simulink model "Serial_Com_Ex"  (R2022b)
settings: Solver=VariableStepAuto  StartTime=0.0  StopTime=10.0  RelTol=1e-3
libraries: etargetslib x4, frdmk64flib x2
settings Model: Creator=samcr  LastModifiedBy=samcr

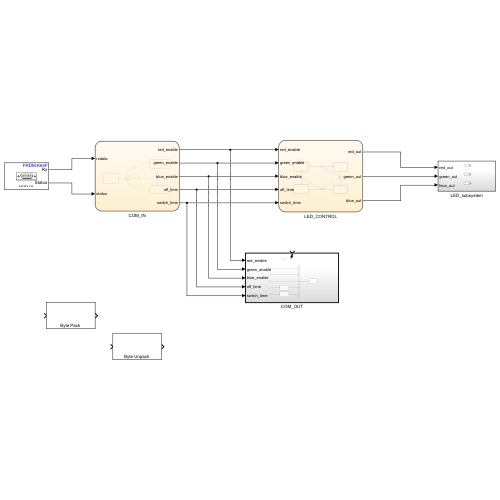
[thumbnail: Simulink's stored preview of the top-level diagram]
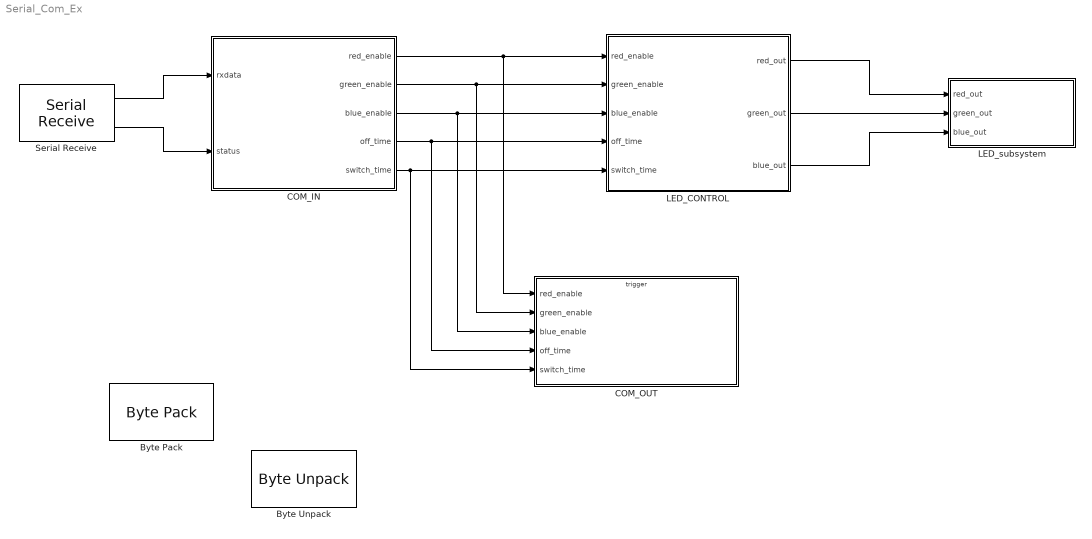
== system Serial_Com_Ex ==
  Byte Pack : etargetslib/Byte Pack  datatypes={'double'}  byteAlign=1
  Byte Unpack : etargetslib/Byte Unpack  dimensions={[1]}  datatypes={'double'}  byteAlign=1
      settings: LibrarySourceBlock=embeddedtargetslib/Host Communication/Byte Unpack
  COM_IN : Stateflow chart  TreatAsAtomicUnit=on
  COM_OUT : Subsystem
  LED_CONTROL : Stateflow chart  TreatAsAtomicUnit=on
  LED_subsystem : Subsystem
  Serial Receive : frdmk64flib/Serial Receive  SCIModule=0  Baudrate=uint32(9600)  Parity=None  StopBits=1  HardwareFlowControl=None  ByteOrder=LittleEndian  DataType=uint8  DataLength=10  BlockingMode=off  OutputStatus=on  SampleTime=-1
  wires:
  Serial Receive/1 -> COM_IN/1(rxdata)
  Serial Receive/2 -> COM_IN/2(status)
  COM_IN/1(red_enable) -> COM_OUT/1(red_enable), LED_CONTROL/1(red_enable)
  COM_IN/2(green_enable) -> COM_OUT/2(green_enable), LED_CONTROL/2(green_enable)
  COM_IN/3(blue_enable) -> COM_OUT/3(blue_enable), LED_CONTROL/3(blue_enable)
  COM_IN/4(off_time) -> COM_OUT/4(off_time), LED_CONTROL/4(off_time)
  COM_IN/5(switch_time) -> LED_CONTROL/5(switch_time), COM_OUT/5(switch_time)
  LED_CONTROL/2(green_out) -> LED_subsystem/2(green_out)
  LED_CONTROL/3(blue_out) -> LED_subsystem/3(blue_out)
  LED_CONTROL/1(red_out) -> LED_subsystem/1(red_out)

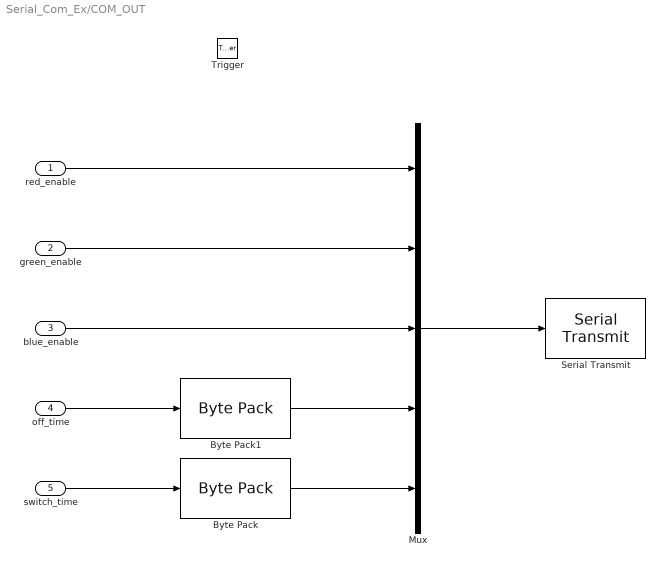
== system Serial_Com_Ex/COM_OUT ==
  red_enable : Inport
  green_enable : Inport  Port=2
  blue_enable : Inport  Port=3
  off_time : Inport  Port=4
  switch_time : Inport  Port=5
  Trigger : TriggerPort  IsSimulinkFunction=on  FunctionName=set_params  VariantControl=(inherit)  PortDimensions=1
  Byte Pack : etargetslib/Byte Pack  datatypes={'double'}  byteAlign=1
  Byte Pack1 : etargetslib/Byte Pack  datatypes={'double'}  byteAlign=1
  Mux : Mux  Inputs=5
  Serial Transmit : frdmk64flib/Serial Transmit  SCIModule=0  Baudrate=uint32(9600)  Parity=None  StopBits=1  HardwareFlowControl=None  ByteOrder=LittleEndian  BlockingMode=on  OutputStatus=off
  wires:
  switch_time/1 -> Byte Pack/1
  off_time/1 -> Byte Pack1/1
  Byte Pack1/1 -> Mux/4
  Byte Pack/1 -> Mux/5
  blue_enable/1 -> Mux/3
  green_enable/1 -> Mux/2
  red_enable/1 -> Mux/1
  Mux/1 -> Serial Transmit/1

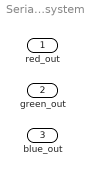
== system Serial_Com_Ex/LED_subsystem ==
  red_out : Inport
  green_out : Inport  Port=2
  blue_out : Inport  Port=3

== stateflow chart Serial_Com_Ex/LED_CONTROL ==
  state OFF
    entry:
    red_out = 0;
    green_out=0;
    blue_out=0;
  state RED_ON
    entry:
    red_out=1;
    green_out = 0;
    blue_out=0;
  note: after(switch_time,msec)
  note: after(switch_time,msec)
  state BLUE_ON
    entry:
    red_out=0;
    green_out = 0;
    blue_out=1;
  state GREEN_ON
    entry:
    red_out=0;
    green_out = 1;
    blue_out=0;
  note: after(switch_time,msec)
  (default) -> OFF
  OFF -> (junction 30) : after(off_time,sec)
  (junction 30) -> RED_ON [order 1] : [red_enable==1]
  (junction 30) -> (junction 31) [order 2]
  (junction 29) -> OFF
  RED_ON -> (junction 31)
  (junction 31) -> (junction 32) [order 2]
  (junction 32) -> (junction 29) [order 2]
  (junction 31) -> GREEN_ON [order 1] : [green_enable==1]
  BLUE_ON -> (junction 29)
  (junction 32) -> BLUE_ON [order 1] : [blue_enable==1]
  GREEN_ON -> (junction 32)
  data: red_enable input; green_enable input; blue_enable input; off_time input; switch_time input; red_out output; green_out output; blue_out output

== stateflow chart Serial_Com_Ex/COM_IN ==
  state SET_PARAM
    entry:
    red_enable= rxdata(3);
    green_enable = rxdata(4);
    blue_enable = rxdata(5);
    off_time = typecast(rxdata(6:9),'single');
    switch_time = typecast(rxdata(10:11),'unit16');
  state INITIAL
    %Set the initial values of the parameters
    entry:
    red_enable = 1;
    green_enable=1;
    blue_enable=0;
    off_time = 0.5; %In Seconds
    switch_time=200;%In Milliseconds
  state STANDBY
  state ECHO_PARAM
    entry:
    send_params();
  SET_PARAM -> STANDBY
  (junction 28) -> SET_PARAM [order 1] : [rxdata(2)==hex2dec('55')]
  (default) -> INITIAL
  (junction 27) -> STANDBY [order 2]
  STANDBY -> (junction 27) : [status==0]
  (junction 27) -> (junction 28) [order 1] : [rxdata(1)==hex2dec('16')]
  (junction 28) -> ECHO_PARAM [order 2] : [rxdata(2)==hex2dec('22')]
  INITIAL -> STANDBY
  ECHO_PARAM -> STANDBY
  data: rxdata input; status input; red_enable output; green_enable output; blue_enable output; off_time output; switch_time output
